simulink model "LQR_Model"  (R2022a)
settings: Solver=VariableStepAuto  StartTime=0.0  StopTime=10.0  RelTol=1e-3
values from neighbouring files (symbols this model uses):
  A = [0 1 0 0 0 0; 0 A22 A23 0 0 0; 0 0 0 1 0 0 ... (first row only)    [LQR1.m]
  B = [0 0; B2 B2; 0 0; B4 B4; 0 0; B6 -B6]    [LQR1.m]
undefined symbols (not defined in the file or in its folder): K
settings Model: Creator=Shiva  LastModifiedBy=Shiva

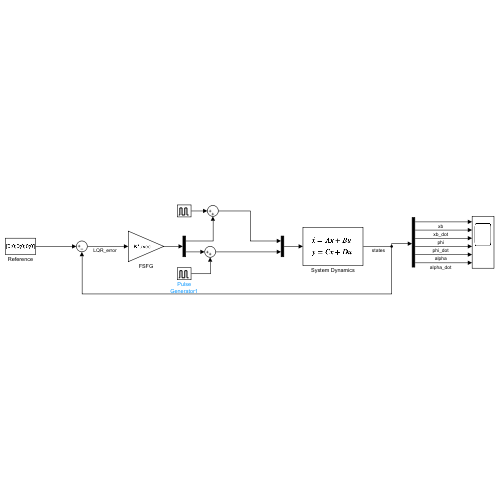
[thumbnail: Simulink's stored preview of the top-level diagram]
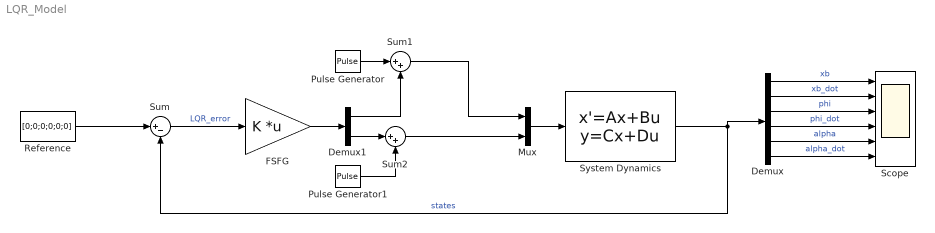
== system LQR_Model ==
  Demux : Demux  Outputs=6
  Demux1 : Demux  Outputs=2
  FSFG : Gain  Gain=K  Multiplication=Matrix(K*u) (u vector)
  Mux : Mux  Inputs=2
  Pulse Generator : DiscretePulseGenerator  PulseType=Time based  Amplitude=0.5  PulseWidth=5
  Pulse Generator1 : DiscretePulseGenerator  PulseType=Time based  Amplitude=0.5  PulseWidth=5
  Reference : Constant  Value=[0;0;0;0;0;0]
  Scope : Scope  NumInputPorts=6
  Sum : Sum  Inputs=|+-
  Sum1 : Sum  Inputs=|++
  Sum2 : Sum  Inputs=|++
  System Dynamics : StateSpace  A=A  B=B  C=eye(6)  D=zeros(6,2)  InitialCondition=0  ParameterTunability=Optimized
  wires:
  Sum/1 -> FSFG/1  "LQR_error"
  System Dynamics/1 -> Demux/1, Sum/2  "states"
  Reference/1 -> Sum/1
  Demux/1 -> Scope/1  "xb"
  Demux/2 -> Scope/2  "xb_dot"
  Demux/3 -> Scope/3  "phi"
  Demux/4 -> Scope/4  "phi_dot"
  Demux/5 -> Scope/5  "alpha"
  Demux/6 -> Scope/6  "alpha_dot"
  FSFG/1 -> Demux1/1
  Demux1/1 -> Sum1/2
  Pulse Generator/1 -> Sum1/1
  Sum1/1 -> Mux/1
  Demux1/2 -> Sum2/1
  Pulse Generator1/1 -> Sum2/2
  Sum2/1 -> Mux/2
  Mux/1 -> System Dynamics/1
